simulink model "SH_core_control"  (R2023b)
settings: configuration reference "ctrl_tsk_conf" (kept outside this file)
undefined symbols (not defined in the file): shuntHarmonicsCorrected, shuntNumHarmonics
settings Model: DataDictionary=fmuGenerationDictionay.sldd  Creator=Veimar  LastModifiedBy=Veimar
settings ConfigSetRef: SourceName=ctrl_tsk_conf

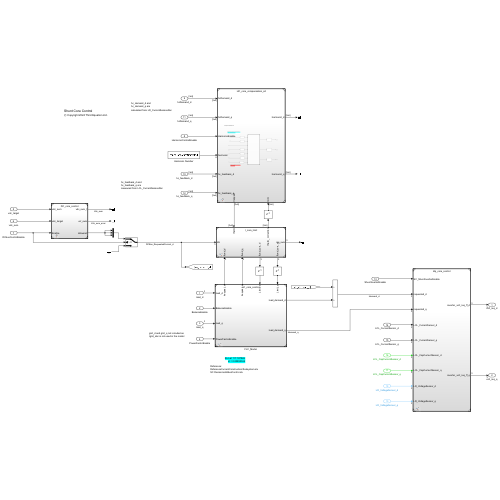
[thumbnail: Simulink's stored preview of the top-level diagram]
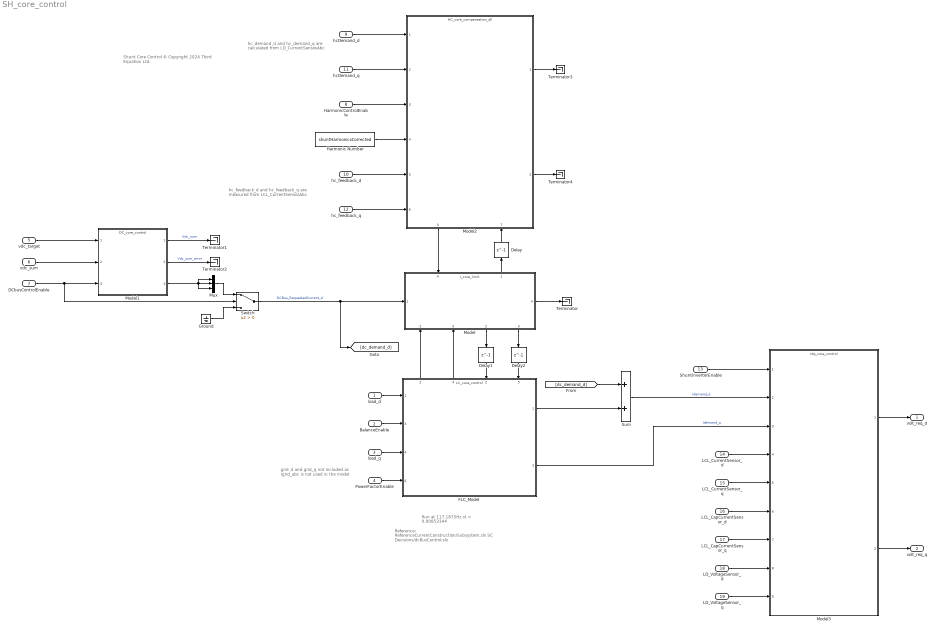
== system SH_core_control ==
  note: hc_feedback_d and
      | hc_feedback_q are
      | measured from LCL_CurrentSensosAbc
  note: Reference:
      | ReferenceCurrentConstruction/Subsystem.slx
      | SC Decisions/dcBusControl.slx
  note: grid_d and grid_q not included as
      | Igrid_abc is not used in the model
  note: Shunt Core Control
      | © Copyright 2024 Third Equation Ltd.
  note: Run at 117.1875Hz
      | st = 0.00853344
  note: hc_demand_d and
      | hc_demand_q are
      | calculated from LD_CurrentSensosAbc
  load_d : Inport  OutDataTypeStr=single  PortDimensions=3
  BalanceEnable : Inport  Port=2  OutDataTypeStr=boolean  PortDimensions=1
  load_q : Inport  Port=3  OutDataTypeStr=single  PortDimensions=3
  PowerFactorEnable : Inport  Port=4  OutDataTypeStr=boolean  PortDimensions=1
  vdc_target : Inport  Port=5  OutDataTypeStr=single  PortDimensions=1
  vdc_sum : Inport  Port=6  OutDataTypeStr=single  PortDimensions=1
  DCbusControlEnable : Inport  Port=7  OutDataTypeStr=boolean  PortDimensions=1
  HarmonicControlEnable : Inport  Port=8  OutDataTypeStr=boolean  PortDimensions=1
  hcDemand_d : Inport  Port=9  OutDataTypeStr=single  PortDimensions=[3 shuntNumHarmonics]
  hc_feedback_d : Inport  Port=10  OutDataTypeStr=single  PortDimensions=[3 shuntNumHarmonics]
  hcDemand_q : Inport  Port=11  OutDataTypeStr=single  PortDimensions=[3 shuntNumHarmonics]
  hc_feedback_q : Inport  Port=12  OutDataTypeStr=single  PortDimensions=[3 shuntNumHarmonics]
  ShuntInverterEnable : Inport  Port=13  OutDataTypeStr=boolean  PortDimensions=1
  LCL_CurrentSensor_d : Inport  Port=14
  LCL_CurrentSensor_q : Inport  Port=15
  LCL_CapCurrentSensor_d : Inport  Port=16
  LCL_CapCurrentSensor_q : Inport  Port=17
  LD_VoltageSensor_d : Inport  Port=18
  LD_VoltageSensor_q : Inport  Port=19
  Delay : Delay  DelayLength=1
  Delay1 : Delay  DelayLength=1
  Delay2 : Delay  DelayLength=1
  FLC_Model : ModelReference  ModelNameDialog=LC_core_control.slx  SimulationMode=Normal  ModelReferenceVersion=1.19
      settings: PortSchema="{\"entries\":[{\"content\":{\"sides\":[{\"content\":{\"connectorIds\":[\"In1\",\"In3\",\"In4\",\"In6\"]},\"type\":\"ConnectorPlacement.EquallySpacedRectSide\",\"uuid\":\"de9eeada-7440-4b08-b2ec-4a7e429c8558\"},{\"content\":{\"connectorIds\":[\"Out1\",\"Out3\"],\"side\":\"RIGHT\"},\"type\":\"ConnectorPlacement.EquallySpacedRectSide\",\"uuid\":\"554e5ea5-630c-4643-a219-0945d0fcd03f\"},{\"content\":{\"connectorIds\":[\"Out2\",\"Out4\",\"In2\",\"In5\"],\"side\":\"TOP\"},\"type\":\"ConnectorPlacement.EquallySpacedRectSide\",\"uuid\":\"a2d436af-8fe7-4db5-8608-b3e61c863679\"}]},\"type\":\"ConnectorPlacement.EquallySpacedConnector\",\"uuid\":\"e9fa697b-8bbc-40c7-ba02-5df4554eaa2f\"}],\"packageUris\":[\"http://schema.mathworks.com/mf0/Connector/R2020b\"],\"version\":\"1.0\"}"
  Ground : Ground
  Harmonic Number : Constant  Value=shuntHarmonicsCorrected  OutDataTypeStr=single
  Model : ModelReference  ModelNameDialog=I_core_limit.slx  SimulationMode=Normal  ModelReferenceVersion=1.74
      settings: PortSchema="{\"entries\":[{\"content\":{\"sides\":[{\"content\":{\"connectorIds\":[\"In1\"]},\"type\":\"ConnectorPlacement.EquallySpacedRectSide\",\"uuid\":\"c776d5dc-1739-4d83-bf20-6e7ac3f81af8\"},{\"content\":{\"connectorIds\":[\"Out4\"],\"side\":\"RIGHT\"},\"type\":\"ConnectorPlacement.EquallySpacedRectSide\",\"uuid\":\"fa4048d2-a318-4ca0-bec8-685a5f092129\"},{\"content\":{\"connectorIds\":[\"In4\",\"Out1\"],\"side\":\"TOP\"},\"type\":\"ConnectorPlacement.EquallySpacedRectSide\",\"uuid\":\"55e25ef1-be30-4043-9c5a-96a8d419b3c3\"},{\"content\":{\"connectorIds\":[\"In2\",\"In3\",\"Out2\",\"Out3\"],\"side\":\"BOTTOM\"},\"type\":\"ConnectorPlacement.EquallySpacedRectSide\",\"uuid\":\"6405c3b5-0f2e-4232-9ea1-6db783170e11\"}]},\"type\":\"ConnectorPlacement.EquallySpacedConnector\",\"uuid\":\"756f9658-6232-4f33-99f5-5ebdafc2b8a1\"}],\"packageUris\":[\"http://schema.mathworks.com/mf0/Connector/R2020b\"],\"version\":\"1.0\"}"
  Model1 : ModelReference  ModelNameDialog=DC_core_control.slx  SimulationMode=Normal  ModelReferenceVersion=1.26
  Model2 : ModelReference  ModelNameDialog=HC_core_compensation_all.slx  SimulationMode=Normal  ModelReferenceVersion=1.42
      settings: PortSchema="{\"entries\":[{\"content\":{\"sides\":[{\"content\":{\"connectorIds\":[\"In1\",\"In2\",\"In3\",\"In4\",\"In5\",\"In6\"]},\"type\":\"ConnectorPlacement.EquallySpacedRectSide\",\"uuid\":\"9f9bd9f4-1593-4b02-bd3d-b3f4ce08cf8a\"},{\"content\":{\"connectorIds\":[\"Out1\",\"Out2\"],\"side\":\"RIGHT\"},\"type\":\"ConnectorPlacement.EquallySpacedRectSide\",\"uuid\":\"e46f214e-0bf7-4013-8eab-5aa080a6ca41\"},{\"content\":{\"side\":\"TOP\"},\"type\":\"ConnectorPlacement.EquallySpacedRectSide\",\"uuid\":\"df5e40bd-2485-42f5-b3f7-7fe017e89dd2\"},{\"content\":{\"connectorIds\":[\"Out3\",\"In7\"],\"side\":\"BOTTOM\"},\"type\":\"ConnectorPlacement.EquallySpacedRectSide\",\"uuid\":\"b702cd5e-9623-49a4-b6dd-056ba0f03c0d\"}]},\"type\":\"ConnectorPlacement.EquallySpacedConnector\",\"uuid\":\"1077302e-2d6f-4243-ad36-8507c375f1a1\"}],\"packageUris\":[\"http://schema.mathworks.com/mf0/Connector/R2020b\"],\"version\":\"1.0\"}"
  Model3 : ModelReference  ModelNameDialog=Idq_core_control.slx  SimulationMode=Normal  ModelReferenceVersion=1.33
  Mux : Mux  Inputs=3
  Sum : Sum
  Switch : Switch  Criteria=u2 > Threshold  SaturateOnIntegerOverflow=off  InputSameDT=off
  Terminator{,1..4} (5 alike) : Terminator
  volt_req_d : Outport  OutDataTypeStr=single  PortDimensions=3
  volt_req_q : Outport  Port=2  OutDataTypeStr=single  PortDimensions=3
  wires:
  load_d/1 -> FLC_Model/1
  BalanceEnable/1 -> FLC_Model/3
  PowerFactorEnable/1 -> FLC_Model/6
  load_q/1 -> FLC_Model/4
  FLC_Model/3 -> Model3/3  "Idemand_q"
  FLC_Model/2 -> Model/2
  FLC_Model/4 -> Model/3
  Model/2 -> Delay1/1
  Model/3 -> Delay2/1
  Model/4 -> Terminator/1
  Model/1 -> Delay/1
  Switch/1 -> Model/1, [dc_demand_d]  "DCBus_RequestedCurrent_d"
  Model1/3 -> Mux/3, Mux/2, Mux/1
  Mux/1 -> Switch/1
  DCbusControlEnable/1 -> Switch/2, Model1/3
  Ground/1 -> Switch/3
  Model1/1 -> Terminator1/1  "Vdc_sum"
  Model1/2 -> Terminator2/1  "Vdc_sum_error"
  vdc_target/1 -> Model1/1
  vdc_sum/1 -> Model1/2
  Harmonic Number/1 -> Model2/4
  HarmonicControlEnable/1 -> Model2/3
  Model2/3 -> Model/4
  hcDemand_d/1 -> Model2/1
  hcDemand_q/1 -> Model2/2
  hc_feedback_d/1 -> Model2/5
  hc_feedback_q/1 -> Model2/6
  Delay/1 -> Model2/7
  Delay1/1 -> FLC_Model/2
  Delay2/1 -> FLC_Model/5
  [dc_demand_d] -> Sum/1
  FLC_Model/1 -> Sum/2
  Sum/1 -> Model3/2  "Idemand_d"
  Model2/1 -> Terminator3/1
  Model2/2 -> Terminator4/1
  ShuntInverterEnable/1 -> Model3/1
  LCL_CurrentSensor_d/1 -> Model3/4
  LCL_CapCurrentSensor_d/1 -> Model3/6
  LD_VoltageSensor_d/1 -> Model3/8
  LCL_CurrentSensor_q/1 -> Model3/5
  LCL_CapCurrentSensor_q/1 -> Model3/7
  LD_VoltageSensor_q/1 -> Model3/9
  Model3/1 -> volt_req_d/1
  Model3/2 -> volt_req_q/1
